simulink model "wlan_phy_tx_pmd"  (Simulink 7.8)
settings: Solver=ode45  StartTime=0.0  StopTime=17e3  RelTol=1e-3
PostLoadFcn:
  | wlan_phy_tx_init
InitFcn:
  | wlan_phy_tx_init
StartFcn:
  | wlan_phy_tx_init
undefined symbols (not defined in the file): gcbh, interleave_16QAM, interleave_64QAM_addr, interleave_bpsk, interleave_QPSK, MAX_NUM_BYTES, MAX_NUM_SC, Mod_Constellation_16QAM, Mod_Constellation_64QAM, Mod_Constellation_BPSK, Mod_Constellation_QPSK, Preamble_IQ, xlBlockLoadCallback, xlGetNormalizedPeriod
libraries: xbsIndex_r4 x1164, xbsEDKLib_r4 x1
(part 3 of 8)

== system wlan_phy_tx_pmd/FFT ==
  Q in : Inport
  I in : Inport  Port=2
  data_in_tvalid : Inport  Port=3
  data_in_tlast : Inport  Port=4
  "Last sym " : Inport  Port=5
  FFT Core : Subsystem
  FFT In : Scope  NumInputPorts=5
      settings: TimeRange=10000  YMin=0~0~-1~-1~0  YMax=1~1~1~1~1
  FFT Last Sym : Scope  NumInputPorts=6
      settings: TimeRange=10000  YMin=0~0~-1~-1~-1~0  YMax=1~80~1~1~1~1  SaveName=ScopeData19
  FFT Out : Scope  NumInputPorts=6
      settings: TimeRange=10000  YMin=0~0~-1~-1~-1~0  YMax=1~80~1~1~1~1
  Gateway Out{,1..13,15..16} (16 alike) : xbsIndex_r4/Gateway Out  inherit_from_input=off  hdl_port=off  timing_constraint=None  locs_specified=off  LOCs={}  UseAsDAC=off  DACChannel='1'  block_type=gatewayout
  Logical : xbsIndex_r4/Logical  logical_function=AND  inputs=2  en=off  latency=0  precision=Full  arith_type=Unsigned  n_bits=16  bin_pt=0  align_bp=on  dbl_ovrd=off  block_type=logical
  S-R Latch2 : Subsystem
  valid only : Subsystem
  valid only1 : Subsystem
  data_in_tready : Outport
  I out : Outport  Port=2
  Q out : Outport  Port=3
  data_out_tvalid : Outport  Port=4
  Last sym : Outport  Port=5
  wires:
  Gateway Out7/1 -> FFT In/5  "tlast"
  valid only/1(Q) -> Gateway Out3/1
  Gateway Out3/1 -> FFT In/4  "valid I data"
  Gateway Out2/1 -> FFT In/3  "I data"
  Gateway Out1/1 -> FFT In/1  "tready"
  Gateway Out/1 -> FFT In/2  "tvalid"
  Gateway Out13/1 -> FFT Out/4  "valid I data"
  Gateway Out12/1 -> FFT Out/3  "I data"
  Gateway Out10/1 -> FFT Out/1  "tvalid"
  valid only1/1(Q) -> Gateway Out13/1
  Gateway Out11/1 -> FFT Out/2  "xk_index"
  "Last sym "/1 -> S-R Latch2/1(S), Gateway Out4/1
  S-R Latch2/1(Q) -> Logical/2, Gateway Out6/1
  Logical/1 -> Last sym/1, Gateway Out15/1, Gateway Out9/1
  [TX_RESET] -> S-R Latch2/2(R), Gateway Out5/1
  Gateway Out15/1 -> FFT Out/6  "Last sym"
  Gateway Out16/1 -> FFT Out/5  "tlast"
  FFT Core/1(data_in_tready) -> data_in_tready/1, Gateway Out1/1, valid only/1(ready)
  FFT Core/2(I out) -> I out/1, Gateway Out12/1, valid only1/1(D)
  FFT Core/3(Q out) -> Q out/1
  Q in/1 -> FFT Core/1(Q in)
  I in/1 -> FFT Core/2(I in), valid only/3(D), Gateway Out2/1
  FFT Core/4(data_out_tvalid) -> data_out_tvalid/1, Gateway Out10/1, valid only1/2(valid)
  data_in_tvalid/1 -> FFT Core/3(data_in_tvalid), Gateway Out/1, valid only/2(valid)
  data_in_tlast/1 -> FFT Core/4(data_in_tlast), Gateway Out7/1
  FFT Core/6(data_out_tlast) -> Gateway Out16/1, Logical/1, Gateway Out8/1
  FFT Core/5(data_xk_index) -> Gateway Out11/1
  Gateway Out4/1 -> FFT Last Sym/1
  Gateway Out5/1 -> FFT Last Sym/2
  Gateway Out6/1 -> FFT Last Sym/3
  Gateway Out8/1 -> FFT Last Sym/4
  Gateway Out9/1 -> FFT Last Sym/5

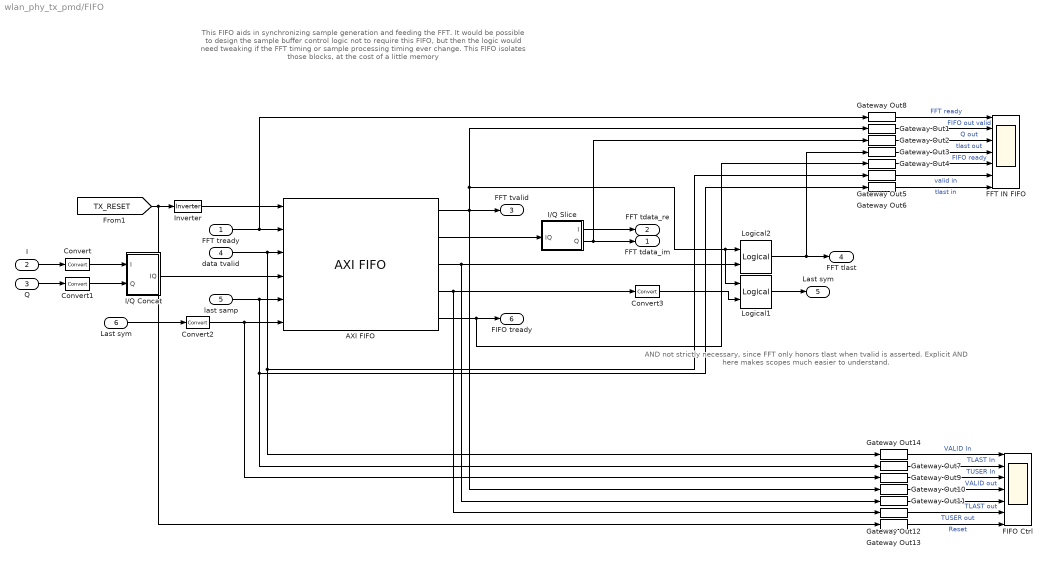
== system wlan_phy_tx_pmd/FIFO ==
  note: AND not strictly necessary, since FFT
      | only honors tlast when tvalid is asserted.
      | Explicit AND here makes scopes
      | much easier to understand.
  note: This FIFO aids in synchronizing sample generation
      | and feeding the FFT. It would be possible to design
      | the sample buffer control logic not to require
      | this FIFO, but then the logic would need tweaking
      | if the FFT timing or sample processing timing
      | ever change. This FIFO isolates those blocks,
      | at the cost of a little memory
  FFT tready : Inport
  I : Inport  Port=2
  Q : Inport  Port=3
  data tvalid : Inport  Port=4
  last samp : Inport  Port=5
  "Last sym " : Inport  Port=6
  AXI FIFO : xbsIndex_r4/AXI FIFO  input_depth_axis=64  actual_fifo_depth_label=66  enable_tdata=on  enable_tdest=off  enable_tstrb=off  enable_tready=on  enable_tid=off  enable_tuser=on  enable_tkeep=off  enable_tlast=on  has_aresetn=on  enable_data_counts_axis=off  fifo_implementation_type_axis=Common Clock Block RAM  trim_axipin_name=on  programmable_full_type_axis=Full  full_threshold_assert_value_axis=0  programmable_empty_type_axis=Empty  empty_threshold_assert_value_axis=1022  block_type=axi_fifo
  Convert : xbsIndex_r4/Convert  gui_display_data_type=Fixed-point  arith_type="Signed  (2's comp)"  n_bits=16  bin_pt=15  float_type=Single  exp_bits=8  fraction_bits=24  quantization=Truncate  overflow=Wrap  en=off  latency=0  dbl_ovrd=off  pipeline=off  block_type=convert
  Convert1 : xbsIndex_r4/Convert  gui_display_data_type=Fixed-point  arith_type="Signed  (2's comp)"  n_bits=16  bin_pt=15  float_type=Single  exp_bits=8  fraction_bits=24  quantization=Truncate  overflow=Wrap  en=off  latency=0  dbl_ovrd=off  pipeline=off  block_type=convert
  Convert2 : xbsIndex_r4/Convert  gui_display_data_type=Fixed-point  arith_type=Unsigned  n_bits=1  bin_pt=0  float_type=Single  exp_bits=8  fraction_bits=24  quantization=Truncate  overflow=Wrap  en=off  latency=0  dbl_ovrd=off  pipeline=off  block_type=convert
  Convert3 : xbsIndex_r4/Convert  gui_display_data_type=Boolean  arith_type=Boolean  n_bits=1  bin_pt=0  float_type=Single  exp_bits=8  fraction_bits=24  quantization=Truncate  overflow=Wrap  en=off  latency=0  dbl_ovrd=off  pipeline=off  block_type=convert
  FFT IN FIFO : Scope  NumInputPorts=7
      settings: TimeRange=30000  YMin=0~0~0~-0.1~0~-0.1~-0.1  YMax=300~300~1~1.1~4000~1.1~1.1  SaveName=ScopeData20
  FIFO Ctrl : Scope  NumInputPorts=7
      settings: TimeRange=30000  YMin=0~0~0~-0.1~-0.1~-0.1~-0.1  YMax=300~300~1~1.1~1.1~1.1~1.1  SaveName=ScopeData21
  Gateway Out{1..14} (14 alike) : xbsIndex_r4/Gateway Out  inherit_from_input=off  hdl_port=off  timing_constraint=None  locs_specified=off  LOCs={}  UseAsDAC=off  DACChannel='1'  block_type=gatewayout
  I/Q Concat : Subsystem
  I/Q Slice : Subsystem
  Inverter : xbsIndex_r4/Inverter  en=off  latency=0  dbl_ovrd=off  block_type=inv
  Logical1 : xbsIndex_r4/Logical  logical_function=AND  inputs=2  en=off  latency=0  precision=Full  arith_type=Unsigned  n_bits=16  bin_pt=0  align_bp=on  dbl_ovrd=off  block_type=logical
  Logical2 : xbsIndex_r4/Logical  logical_function=AND  inputs=2  en=off  latency=0  precision=Full  arith_type=Unsigned  n_bits=16  bin_pt=0  align_bp=on  dbl_ovrd=off  block_type=logical
  FFT tdata_im : Outport
  FFT tdata_re : Outport  Port=2
  FFT tvalid : Outport  Port=3
  FFT tlast : Outport  Port=4
  Last sym : Outport  Port=5
  FIFO tready : Outport  Port=6
  wires:
  FFT tready/1 -> Gateway Out8/1, AXI FIFO/2
  data tvalid/1 -> AXI FIFO/3, Gateway Out5/1, Gateway Out14/1
  last samp/1 -> AXI FIFO/5, Gateway Out6/1, Gateway Out7/1
  I/1 -> Convert/1
  Q/1 -> Convert1/1
  I/Q Concat/1(IQ) -> AXI FIFO/4
  [TX_RESET] -> Inverter/1, Gateway Out13/1
  Inverter/1 -> AXI FIFO/1
  Convert/1 -> I/Q Concat/1(I)
  Convert1/1 -> I/Q Concat/2(Q)
  "Last sym "/1 -> Convert2/1
  AXI FIFO/5 -> FIFO tready/1, Gateway Out4/1
  AXI FIFO/2 -> I/Q Slice/1(IQ)
  AXI FIFO/1 -> FFT tvalid/1, Gateway Out1/1, Logical2/1, Logical1/1, Gateway Out10/1
  AXI FIFO/3 -> Logical2/2, Gateway Out11/1
  Gateway Out8/1 -> FFT IN FIFO/1  "FFT ready"
  I/Q Slice/1(I) -> FFT tdata_re/1
  I/Q Slice/2(Q) -> FFT tdata_im/1, Gateway Out2/1
  Gateway Out1/1 -> FFT IN FIFO/2  "FIFO out valid"
  Gateway Out2/1 -> FFT IN FIFO/3  "Q out"
  Gateway Out3/1 -> FFT IN FIFO/4  "tlast out"
  Gateway Out4/1 -> FFT IN FIFO/5  "FIFO ready"
  Gateway Out5/1 -> FFT IN FIFO/6  "valid in"
  Gateway Out6/1 -> FFT IN FIFO/7  "tlast in"
  Logical2/1 -> FFT tlast/1, Gateway Out3/1
  AXI FIFO/4 -> Gateway Out12/1, Convert3/1
  Convert2/1 -> AXI FIFO/6, Gateway Out9/1
  Gateway Out14/1 -> FIFO Ctrl/1  "VALID In"
  Gateway Out7/1 -> FIFO Ctrl/2  "TLAST In"
  Gateway Out9/1 -> FIFO Ctrl/3  "TUSER In"
  Gateway Out10/1 -> FIFO Ctrl/4  "VALID out"
  Gateway Out11/1 -> FIFO Ctrl/5  "TLAST out"
  Gateway Out12/1 -> FIFO Ctrl/6  "TUSER out"
  Gateway Out13/1 -> FIFO Ctrl/7  "Reset"
  Logical1/1 -> Last sym/1
  Convert3/1 -> Logical1/2

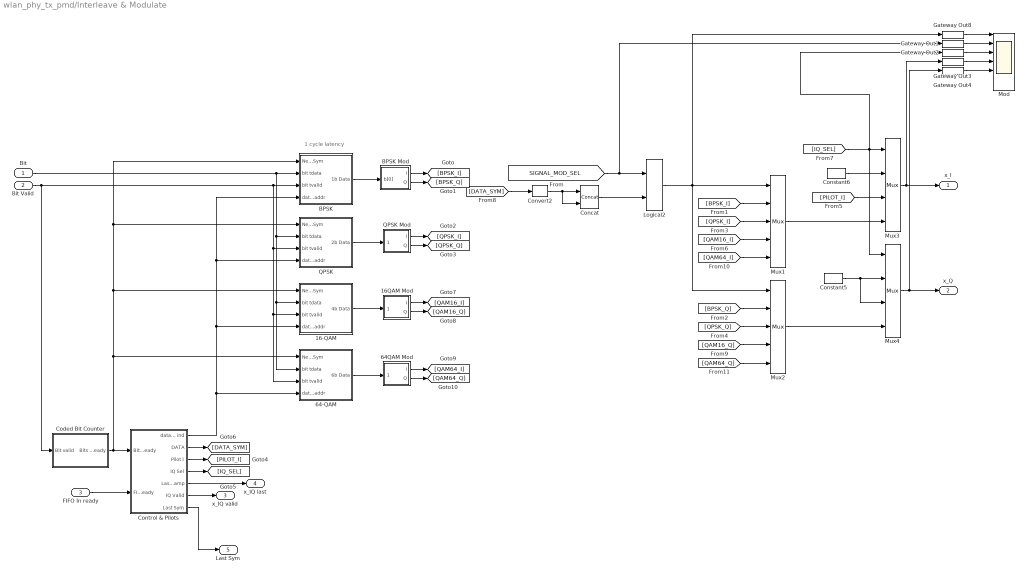
== system wlan_phy_tx_pmd/Interleave & Modulate ==
  note: 1 cycle latency
  Bit : Inport
  Bit Valid : Inport  Port=2
  FIFO In ready : Inport  Port=3
  16-QAM : Subsystem
  16QAM Mod : Subsystem
  64-QAM : Subsystem
  64QAM Mod : Subsystem
  BPSK : Subsystem
  BPSK Mod : Subsystem
  Coded Bit Counter : Subsystem
  Concat : xbsIndex_r4/Concat  num_inputs=2  dbl_ovrd=off  block_type=concat
  Constant5 : xbsIndex_r4/Constant  const=0  gui_display_data_type=Fixed-point  arith_type=Signed (2's comp)  n_bits=12  bin_pt=11  preci_type=Single  exp_width=8  frac_width=24  explicit_period=off  period=1  equ=P=C  opselect=C  inp2=PCIN>>17  opr=+  inp1=P  carry=CIN  dbl_ovrd=off  block_type=constant
  Constant6 : xbsIndex_r4/Constant  const=0  gui_display_data_type=Fixed-point  arith_type=Signed (2's comp)  n_bits=12  bin_pt=11  preci_type=Single  exp_width=8  frac_width=24  explicit_period=off  period=1  equ=P=C  opselect=C  inp2=PCIN>>17  opr=+  inp1=P  carry=CIN  dbl_ovrd=off  block_type=constant
  Control & Pilots : Subsystem
  Convert2 : xbsIndex_r4/Convert  gui_display_data_type=Fixed-point  arith_type=Unsigned  n_bits=1  bin_pt=0  float_type=Single  exp_bits=8  fraction_bits=24  quantization=Truncate  overflow=Wrap  en=off  latency=0  dbl_ovrd=off  pipeline=off  block_type=convert
  Gateway Out{1..4,8} (5 alike) : xbsIndex_r4/Gateway Out  inherit_from_input=off  hdl_port=off  timing_constraint=None  locs_specified=off  LOCs={}  UseAsDAC=off  DACChannel='1'  block_type=gatewayout
  Logical2 : xbsIndex_r4/Logical  logical_function=AND  inputs=2  en=off  latency=0  precision=Full  arith_type=Unsigned  n_bits=16  bin_pt=0  align_bp=on  dbl_ovrd=off  block_type=logical
  "Mod " : Scope  NumInputPorts=7
      settings: TimeRange=10000  YMin=0~0~0~-2~0~-0.1~-0.1  YMax=300~300~1~2~4000~1.1~1.1  SaveName=ScopeData7
  Mux1 : xbsIndex_r4/Mux  inputs=4  en=off  latency=0  precision=Full  arith_type=Unsigned  n_bits=16  bin_pt=14  quantization=Truncate  overflow=Wrap  dbl_ovrd=off  block_type=mux
  Mux2 : xbsIndex_r4/Mux  inputs=4  en=off  latency=0  precision=Full  arith_type=Unsigned  n_bits=16  bin_pt=14  quantization=Truncate  overflow=Wrap  dbl_ovrd=off  block_type=mux
  Mux3 : xbsIndex_r4/Mux  inputs=3  en=off  latency=0  precision=Full  arith_type=Unsigned  n_bits=16  bin_pt=14  quantization=Truncate  overflow=Wrap  dbl_ovrd=off  block_type=mux
  Mux4 : xbsIndex_r4/Mux  inputs=3  en=off  latency=0  precision=Full  arith_type=Unsigned  n_bits=16  bin_pt=14  quantization=Truncate  overflow=Wrap  dbl_ovrd=off  block_type=mux
  QPSK : Subsystem
  QPSK Mod : Subsystem
  x_I : Outport
  x_Q : Outport  Port=2
  x_IQ valid : Outport  Port=3
  x_IQ last : Outport  Port=4
  Last Sym : Outport  Port=5
  wires:
  Convert2/1 -> Concat/2, Concat/1
  [SIGNAL_MOD_SEL] -> Logical2/1, Gateway Out1/1
  Concat/1 -> Logical2/2
  Bit/1 -> BPSK/2("bit tdata "), QPSK/2("bit tdata "), 16-QAM/2("bit tdata "), 64-QAM/2("bit tdata ")
  Bit Valid/1 -> BPSK/3("bit tvalid "), QPSK/3("bit tvalid "), 16-QAM/3("bit tvalid "), 64-QAM/3("bit tvalid "), Coded Bit Counter/1(Bit valid)
  BPSK/1(1b Data) -> BPSK Mod/1(b[0])
  QPSK/1(2b Data) -> QPSK Mod/1(b[1:0])
  [QAM64_I] -> Mux1/5
  [QAM64_Q] -> Mux2/5
  BPSK Mod/1(I) -> [BPSK_I]
  BPSK Mod/2(Q) -> [BPSK_Q]
  QPSK Mod/1(I) -> [QPSK_I]
  QPSK Mod/2(Q) -> [QPSK_Q]
  [BPSK_Q] -> Mux2/2
  [BPSK_I] -> Mux1/2
  [QPSK_Q] -> Mux2/3
  Logical2/1 -> Mux1/1, Mux2/1, Gateway Out8/1
  [QPSK_I] -> Mux1/3
  Constant5/1 -> Mux4/2, Mux4/3
  Constant6/1 -> Mux3/2
  Control & Pilots/3(Pilot I) -> [PILOT_I]
  [PILOT_I] -> Mux3/3
  Mux1/1 -> Mux3/4
  Mux2/1 -> Mux4/4
  Mux3/1 -> x_I/1, Gateway Out3/1
  Mux4/1 -> x_Q/1, Gateway Out4/1
  Control & Pilots/4(IQ Sel) -> [IQ_SEL]
  [IQ_SEL] -> Mux3/1, Mux4/1, Gateway Out2/1
  Control & Pilots/5(Last Samp) -> x_IQ last/1
  Control & Pilots/6(IQ Valid) -> x_IQ valid/1
  [DATA_SYM] -> Convert2/1
  Control & Pilots/2(DATA) -> [DATA_SYM]
  Gateway Out8/1 -> "Mod "/1
  Gateway Out1/1 -> "Mod "/2
  Gateway Out2/1 -> "Mod "/3
  Gateway Out3/1 -> "Mod "/4
  Gateway Out4/1 -> "Mod "/5
  Coded Bit Counter/1(Bits Ready) -> Control & Pilots/1(Bits Ready), BPSK/1(New Sym), QPSK/1(New Sym), 16-QAM/1(New Sym), 64-QAM/1(New Sym)
  Control & Pilots/7(" Last Sym") -> Last Sym/1
  FIFO In ready/1 -> Control & Pilots/2(FIFO Ready)
  16-QAM/1(4b Data) -> 16QAM Mod/1(b[3:0])
  16QAM Mod/1(I) -> [QAM16_I]
  16QAM Mod/2(Q) -> [QAM16_Q]
  [QAM16_I] -> Mux1/4
  [QAM16_Q] -> Mux2/4
  Control & Pilots/1(data sym ind) -> 64-QAM/4(data sym addr), 16-QAM/4(data sym addr), QPSK/4(data sym addr), BPSK/4(data sym addr)
  64QAM Mod/1(I) -> [QAM64_I]
  64QAM Mod/2(Q) -> [QAM64_Q]
  64-QAM/1(6b Data) -> 64QAM Mod/1(b[5:0])

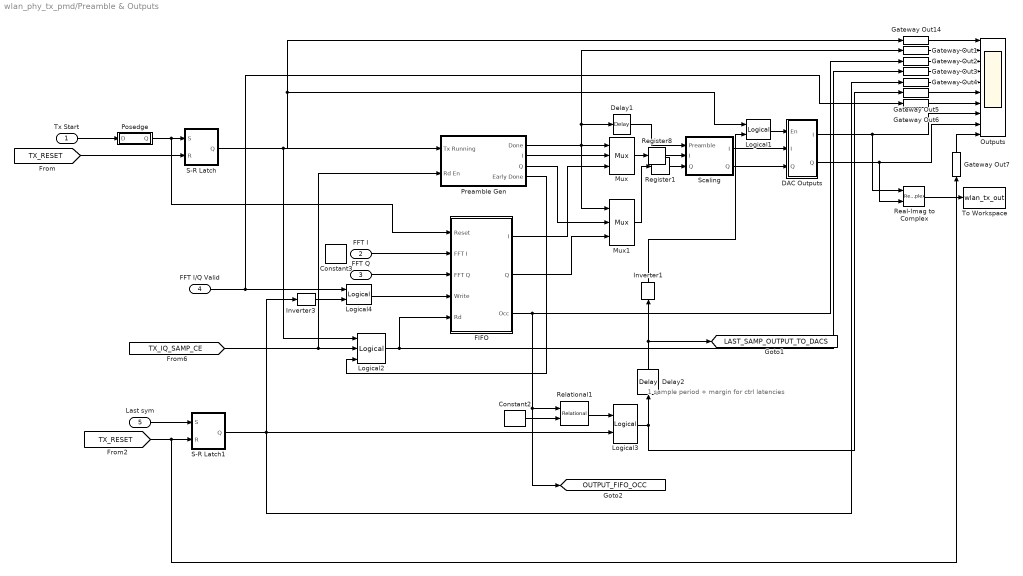
== system wlan_phy_tx_pmd/Preamble & Outputs ==
  note: 1 sample period + margin
      | for ctrl latencies
  Tx Start : Inport
  FFT I : Inport  Port=2
  FFT Q : Inport  Port=3
  FFT I/Q Valid : Inport  Port=4
  Last sym : Inport  Port=5
  Constant2 : xbsIndex_r4/Constant  const=0  gui_display_data_type=Fixed-point  arith_type=Unsigned  n_bits=1  bin_pt=0  preci_type=Single  exp_width=8  frac_width=24  explicit_period=off  period=1  equ=P=C  opselect=C  inp2=PCIN>>17  opr=+  inp1=P  carry=CIN  dbl_ovrd=off  block_type=constant
  Constant3 : xbsIndex_r4/Constant  const=-1  gui_display_data_type=Fixed-point  arith_type=Signed (2's comp)  n_bits=16  bin_pt=15  preci_type=Single  exp_width=8  frac_width=24  explicit_period=on  period=1  equ=P=C  opselect=C  inp2=PCIN>>17  opr=+  inp1=P  carry=CIN  dbl_ovrd=off  block_type=constant
  DAC Outputs : Subsystem
  Delay1 : xbsIndex_r4/Delay  rst=off  infoeditControl=Selection of Reset will increase slice count due to use of real FFs and instead of SRLs  en=off  latency=1  dbl_ovrd=off  reg_retiming=off  block_type=delay
  Delay2 : xbsIndex_r4/Delay  rst=off  infoeditControl=Selection of Reset will increase slice count due to use of real FFs and instead of SRLs  en=off  latency=12  dbl_ovrd=off  reg_retiming=off  block_type=delay
  FIFO : Subsystem
  Gateway Out{1..7,14} (8 alike) : xbsIndex_r4/Gateway Out  inherit_from_input=off  hdl_port=off  timing_constraint=None  locs_specified=off  LOCs={}  UseAsDAC=off  DACChannel='1'  block_type=gatewayout
  Inverter1 : xbsIndex_r4/Inverter  en=off  latency=0  dbl_ovrd=off  block_type=inv
      settings: xl_area=[0 0 0 0 0 0 0]  block_version=VER_STRING_GOES_HERE
  Inverter3 : xbsIndex_r4/Inverter  en=off  latency=0  dbl_ovrd=off  block_type=inv
      settings: xl_area=[0 0 0 0 0 0 0]  block_version=VER_STRING_GOES_HERE
  Logical1 : xbsIndex_r4/Logical  logical_function=AND  inputs=2  en=off  latency=0  precision=Full  arith_type=Unsigned  n_bits=16  bin_pt=0  align_bp=on  dbl_ovrd=off  block_type=logical
  Logical2 : xbsIndex_r4/Logical  logical_function=AND  inputs=3  en=off  latency=0  precision=Full  arith_type=Unsigned  n_bits=16  bin_pt=0  align_bp=on  dbl_ovrd=off  block_type=logical
  Logical3 : xbsIndex_r4/Logical  logical_function=AND  inputs=2  en=off  latency=0  precision=Full  arith_type=Unsigned  n_bits=16  bin_pt=0  align_bp=on  dbl_ovrd=off  block_type=logical
  Logical4 : xbsIndex_r4/Logical  logical_function=AND  inputs=2  en=off  latency=0  precision=Full  arith_type=Unsigned  n_bits=16  bin_pt=0  align_bp=on  dbl_ovrd=off  block_type=logical
  Mux : xbsIndex_r4/Mux  inputs=2  en=off  latency=0  precision=Full  arith_type=Unsigned  n_bits=16  bin_pt=14  quantization=Truncate  overflow=Wrap  dbl_ovrd=off  block_type=mux
  Mux1 : xbsIndex_r4/Mux  inputs=2  en=off  latency=0  precision=Full  arith_type=Unsigned  n_bits=16  bin_pt=14  quantization=Truncate  overflow=Wrap  dbl_ovrd=off  block_type=mux
  Outputs : Scope  NumInputPorts=10
      settings: TimeRange=12000  YMin=0~0~0~0~0~0~0~-1~-0.5~0  YMax=1~1~200~1~1~1~1~1~1~1  SaveName=ScopeData20
  Posedge : Subsystem
  Preamble Gen : Subsystem
  Real-Imag to Complex : RealImagToComplex
  Register1 : xbsIndex_r4/Register  init=0  rst=off  en=off  dbl_ovrd=off  block_type=register
  Register8 : xbsIndex_r4/Register  init=0  rst=off  en=off  dbl_ovrd=off  block_type=register
  Relational1 : xbsIndex_r4/Relational  mode=a=b  en=off  latency=0  dbl_ovrd=off  block_type=relational
  S-R Latch : Subsystem
  S-R Latch1 : Subsystem
  Scaling : Subsystem
  To Workspace : ToWorkspace  VariableName=wlan_tx_out  SampleTime=-1  SaveFormat=Array
      settings: Decimation=8
  tag scope: LAST_SAMP_OUTPUT_TO_DACS=global, OUTPUT_FIFO_OCC=global
  wires:
  Logical2/1 -> FIFO/5(Rd), Gateway Out3/1
  Posedge/1(Q) -> S-R Latch/1(S), FIFO/1(Reset)
  Tx Start/1 -> Posedge/1(D)
  [TX_RESET] -> S-R Latch/2(R)
  S-R Latch/1(Q) -> Logical2/1, Gateway Out14/1, Logical1/1, Preamble Gen/1(Tx Running)
  [TX_IQ_SAMP_CE] -> Logical2/2, Preamble Gen/2(Rd En)
  FFT Q/1 -> FIFO/3(FFT Q)
  Logical4/1 -> FIFO/4(Write)
  FIFO/3(" Occ") -> Relational1/1, [OUTPUT_FIFO_OCC], Gateway Out2/1
  Constant2/1 -> Relational1/2
  Relational1/1 -> Logical3/1
  Last sym/1 -> S-R Latch1/1(S)
  S-R Latch1/1(Q) -> Inverter3/1, Logical3/2, Gateway Out4/1
  Logical3/1 -> Gateway Out5/1, Delay2/1
  [TX_RESET] -> S-R Latch1/2(R), Gateway Out7/1
  Inverter3/1 -> Logical4/2
  FFT I/Q Valid/1 -> Logical4/1, Gateway Out6/1
  FIFO/1(" I") -> Mux/3
  DAC Outputs/1(" I") -> Real-Imag to Complex/1, Outputs/8
  Preamble Gen/2(I) -> Mux/2
  Gateway Out14/1 -> Outputs/1
  Gateway Out1/1 -> Outputs/2
  Gateway Out2/1 -> Outputs/3
  Gateway Out3/1 -> Outputs/4
  Gateway Out4/1 -> Outputs/5
  Gateway Out5/1 -> Outputs/6
  Preamble Gen/1(Done) -> Mux/1, Delay1/1, Gateway Out1/1, Mux1/1
  Real-Imag to Complex/1 -> To Workspace/1
  DAC Outputs/2(" Q") -> Real-Imag to Complex/2, Outputs/9
  Mux/1 -> Register8/1
  Mux1/1 -> Register1/1
  Preamble Gen/3(Q) -> Mux1/2
  FIFO/2(" Q") -> Mux1/3
  Scaling/1(" I") -> DAC Outputs/2(I)
  Scaling/2(" Q") -> DAC Outputs/3(Q)
  Delay1/1 -> Scaling/1(Preamble)
  Logical1/1 -> DAC Outputs/1(En)
  Inverter1/1 -> Logical1/2
  Delay2/1 -> Inverter1/1, [LAST_SAMP_OUTPUT_TO_DACS]
  Gateway Out6/1 -> Outputs/7
  Preamble Gen/4(Early Done) -> Logical2/3
  Gateway Out7/1 -> Outputs/10
  FFT I/1 -> FIFO/2(FFT I)
  Register8/1 -> Scaling/2(I)
  Register1/1 -> Scaling/3(Q)

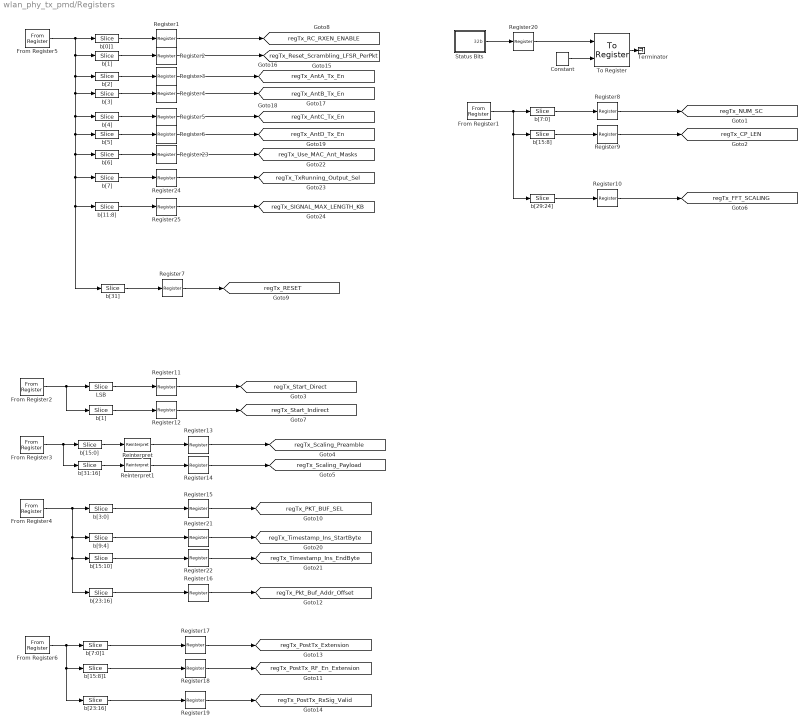
== system wlan_phy_tx_pmd/Registers ==
  Constant : xbsIndex_r4/Constant  const=1  gui_display_data_type=Boolean  arith_type=Boolean  n_bits=16  bin_pt=14  preci_type=Single  exp_width=8  frac_width=24  explicit_period=on  period=1  equ=P=C  opselect=C  inp2=PCIN>>17  opr=+  inp1=P  carry=CIN  dbl_ovrd=off  block_type=constant
  From Register1 : xbsIndex_r4/From Register  shared_memory_name='FFT_Config'  init=REG_TX_FFT_Config  period=1  ownership=Locally owned and initialized  gui_display_data_type=Fixed-point  arith_type=Unsigned  n_bits=32  bin_pt=0  preci_type=Single  dbl_ovrd=off  block_type=fromreg
      settings: AttributesFormatString=<< %<shared_memory_name> >>  infoedit="Register block that reads data to a shared memory register.  Delay of one sample period."
  From Register2 : xbsIndex_r4/From Register  shared_memory_name='TX_START'  init=0  period=1  ownership=Locally owned and initialized  gui_display_data_type=Fixed-point  arith_type=Unsigned  n_bits=32  bin_pt=0  preci_type=Single  dbl_ovrd=off  block_type=fromreg
      settings: AttributesFormatString=<< %<shared_memory_name> >>  infoedit="Register block that reads data to a shared memory register.  Delay of one sample period."
  From Register3 : xbsIndex_r4/From Register  shared_memory_name='Output_Scaling'  init=REG_TX_Output_Scaling  period=1  ownership=Locally owned and initialized  gui_display_data_type=Fixed-point  arith_type=Unsigned  n_bits=32  bin_pt=0  preci_type=Single  dbl_ovrd=off  block_type=fromreg
      settings: AttributesFormatString=<< %<shared_memory_name> >>  infoedit="Register block that reads data to a shared memory register.  Delay of one sample period."
  From Register4 : xbsIndex_r4/From Register  shared_memory_name='PKT_BUF_SEL'  init=REG_TX_PKT_BUF_SEL  period=1  ownership=Locally owned and initialized  gui_display_data_type=Fixed-point  arith_type=Unsigned  n_bits=32  bin_pt=0  preci_type=Single  dbl_ovrd=off  block_type=fromreg
      settings: AttributesFormatString=<< %<shared_memory_name> >>  infoedit="Register block that reads data to a shared memory register.  Delay of one sample period."
  From Register5 : xbsIndex_r4/From Register  shared_memory_name='Config'  init=REG_TX_Config  period=1  ownership=Locally owned and initialized  gui_display_data_type=Fixed-point  arith_type=Unsigned  n_bits=32  bin_pt=0  preci_type=Single  dbl_ovrd=off  block_type=fromreg
      settings: AttributesFormatString=<< %<shared_memory_name> >>  infoedit="Register block that reads data to a shared memory register.  Delay of one sample period."
  From Register6 : xbsIndex_r4/From Register  shared_memory_name='Timing'  init=REG_Tx_Timing  period=1  ownership=Locally owned and initialized  gui_display_data_type=Fixed-point  arith_type=Unsigned  n_bits=32  bin_pt=0  preci_type=Single  dbl_ovrd=off  block_type=fromreg
      settings: AttributesFormatString=<< %<shared_memory_name> >>  infoedit="Register block that reads data to a shared memory register.  Delay of one sample period."
  LSB : xbsIndex_r4/Slice  nbits=1  boolean_output=off  mode=Lower Bit Location + Width  bit1=0  base1=MSB of Input  bit0=0  base0=LSB of Input  dbl_ovrd=off  block_type=slice
      settings: block_version=VER_STRING_GOES_HERE
  Register{1..25} (25 alike) : xbsIndex_r4/Register  init=0  rst=off  en=off  dbl_ovrd=off  block_type=register
  Reinterpret : xbsIndex_r4/Reinterpret  force_arith_type=on  arith_type=Unsigned  force_bin_pt=on  bin_pt=12  block_type=reinterpret
  Reinterpret1 : xbsIndex_r4/Reinterpret  force_arith_type=on  arith_type=Unsigned  force_bin_pt=on  bin_pt=12  block_type=reinterpret
  Status Bits : Subsystem
  Terminator : Terminator
  To Register : xbsIndex_r4/To Register  shared_memory_name='STATUS'  init=0  ownership=Locally owned and initialized  explicit_data_type=on  gui_display_data_type=Fixed-point  arith_type=Unsigned  n_bits=32  bin_pt=0  preci_type=Single  dbl_ovrd=off  block_type=toreg
      settings: AttributesFormatString=<< %<shared_memory_name> >>  infoedit="Register block that writes data to a shared memory register.  Delay of one sample period."
  b[0]1 : xbsIndex_r4/Slice  nbits=1  boolean_output=off  mode=Lower Bit Location + Width  bit1=0  base1=MSB of Input  bit0=0  base0=LSB of Input  dbl_ovrd=off  block_type=slice
      settings: block_version=VER_STRING_GOES_HERE
  b[11:8] : xbsIndex_r4/Slice  nbits=4  boolean_output=off  mode=Lower Bit Location + Width  bit1=0  base1=MSB of Input  bit0=8  base0=LSB of Input  dbl_ovrd=off  block_type=slice
      settings: block_version=VER_STRING_GOES_HERE
  b[15:0] : xbsIndex_r4/Slice  nbits=16  boolean_output=off  mode=Lower Bit Location + Width  bit1=0  base1=MSB of Input  bit0=0  base0=LSB of Input  dbl_ovrd=off  block_type=slice
      settings: block_version=VER_STRING_GOES_HERE
  b[15:10] : xbsIndex_r4/Slice  nbits=6  boolean_output=off  mode=Lower Bit Location + Width  bit1=0  base1=MSB of Input  bit0=10  base0=LSB of Input  dbl_ovrd=off  block_type=slice
      settings: block_version=VER_STRING_GOES_HERE
  b[15:8] : xbsIndex_r4/Slice  nbits=8  boolean_output=off  mode=Lower Bit Location + Width  bit1=0  base1=MSB of Input  bit0=8  base0=LSB of Input  dbl_ovrd=off  block_type=slice
      settings: block_version=VER_STRING_GOES_HERE
  b[15:8]1 : xbsIndex_r4/Slice  nbits=8  boolean_output=off  mode=Lower Bit Location + Width  bit1=0  base1=MSB of Input  bit0=8  base0=LSB of Input  dbl_ovrd=off  block_type=slice
      settings: block_version=VER_STRING_GOES_HERE
  b[1] : xbsIndex_r4/Slice  nbits=1  boolean_output=on  mode=Lower Bit Location + Width  bit1=0  base1=MSB of Input  bit0=1  base0=LSB of Input  dbl_ovrd=off  block_type=slice
      settings: block_version=VER_STRING_GOES_HERE
  "b[1]  " : xbsIndex_r4/Slice  nbits=1  boolean_output=off  mode=Lower Bit Location + Width  bit1=0  base1=MSB of Input  bit0=1  base0=LSB of Input  dbl_ovrd=off  block_type=slice
      settings: block_version=VER_STRING_GOES_HERE
  b[23:16] : xbsIndex_r4/Slice  nbits=8  boolean_output=off  mode=Lower Bit Location + Width  bit1=0  base1=MSB of Input  bit0=16  base0=LSB of Input  dbl_ovrd=off  block_type=slice
      settings: block_version=VER_STRING_GOES_HERE
  "b[23:16] " : xbsIndex_r4/Slice  nbits=8  boolean_output=off  mode=Lower Bit Location + Width  bit1=0  base1=MSB of Input  bit0=16  base0=LSB of Input  dbl_ovrd=off  block_type=slice
      settings: block_version=VER_STRING_GOES_HERE
  b[29:24] : xbsIndex_r4/Slice  nbits=6  boolean_output=off  mode=Lower Bit Location + Width  bit1=0  base1=MSB of Input  bit0=24  base0=LSB of Input  dbl_ovrd=off  block_type=slice
      settings: block_version=VER_STRING_GOES_HERE
  b[2] : xbsIndex_r4/Slice  nbits=1  boolean_output=on  mode=Lower Bit Location + Width  bit1=0  base1=MSB of Input  bit0=2  base0=LSB of Input  dbl_ovrd=off  block_type=slice
      settings: block_version=VER_STRING_GOES_HERE
  b[31:16] : xbsIndex_r4/Slice  nbits=16  boolean_output=off  mode=Lower Bit Location + Width  bit1=0  base1=MSB of Input  bit0=16  base0=LSB of Input  dbl_ovrd=off  block_type=slice
      settings: block_version=VER_STRING_GOES_HERE
  b[31] : xbsIndex_r4/Slice  nbits=1  boolean_output=off  mode=Lower Bit Location + Width  bit1=0  base1=MSB of Input  bit0=31  base0=LSB of Input  dbl_ovrd=off  block_type=slice
      settings: block_version=VER_STRING_GOES_HERE
  b[3:0] : xbsIndex_r4/Slice  nbits=4  boolean_output=off  mode=Lower Bit Location + Width  bit1=0  base1=MSB of Input  bit0=0  base0=LSB of Input  dbl_ovrd=off  block_type=slice
      settings: block_version=VER_STRING_GOES_HERE
  b[3] : xbsIndex_r4/Slice  nbits=1  boolean_output=on  mode=Lower Bit Location + Width  bit1=0  base1=MSB of Input  bit0=3  base0=LSB of Input  dbl_ovrd=off  block_type=slice
      settings: block_version=VER_STRING_GOES_HERE
  b[4] : xbsIndex_r4/Slice  nbits=1  boolean_output=on  mode=Lower Bit Location + Width  bit1=0  base1=MSB of Input  bit0=4  base0=LSB of Input  dbl_ovrd=off  block_type=slice
      settings: block_version=VER_STRING_GOES_HERE
  b[5] : xbsIndex_r4/Slice  nbits=1  boolean_output=on  mode=Lower Bit Location + Width  bit1=0  base1=MSB of Input  bit0=5  base0=LSB of Input  dbl_ovrd=off  block_type=slice
      settings: block_version=VER_STRING_GOES_HERE
  b[6] : xbsIndex_r4/Slice  nbits=1  boolean_output=on  mode=Lower Bit Location + Width  bit1=0  base1=MSB of Input  bit0=6  base0=LSB of Input  dbl_ovrd=off  block_type=slice
      settings: block_version=VER_STRING_GOES_HERE
  b[7:0] : xbsIndex_r4/Slice  nbits=8  boolean_output=off  mode=Lower Bit Location + Width  bit1=0  base1=MSB of Input  bit0=0  base0=LSB of Input  dbl_ovrd=off  block_type=slice
      settings: block_version=VER_STRING_GOES_HERE
  b[7:0]1 : xbsIndex_r4/Slice  nbits=8  boolean_output=off  mode=Lower Bit Location + Width  bit1=0  base1=MSB of Input  bit0=0  base0=LSB of Input  dbl_ovrd=off  block_type=slice
      settings: block_version=VER_STRING_GOES_HERE
  b[7] : xbsIndex_r4/Slice  nbits=1  boolean_output=on  mode=Lower Bit Location + Width  bit1=0  base1=MSB of Input  bit0=7  base0=LSB of Input  dbl_ovrd=off  block_type=slice
      settings: block_version=VER_STRING_GOES_HERE
  b[9:4] : xbsIndex_r4/Slice  nbits=6  boolean_output=off  mode=Lower Bit Location + Width  bit1=0  base1=MSB of Input  bit0=4  base0=LSB of Input  dbl_ovrd=off  block_type=slice
      settings: block_version=VER_STRING_GOES_HERE
  tag scope: regTx_AntA_Tx_En=global, regTx_AntB_Tx_En=global, regTx_AntC_Tx_En=global, regTx_AntD_Tx_En=global, regTx_CP_LEN=global, regTx_FFT_SCALING=global, regTx_NUM_SC=global, regTx_PKT_BUF_SEL=global, regTx_Pkt_Buf_Addr_Offset=global, regTx_PostTx_Extension=global, regTx_PostTx_RF_En_Extension=global, regTx_PostTx_RxSig_Valid=global, regTx_RC_RXEN_ENABLE=global, regTx_RESET=global, regTx_Reset_Scrambling_LFSR_PerPkt=global, regTx_SIGNAL_MAX_LENGTH_KB=global, regTx_Scaling_Payload=global, regTx_Scaling_Preamble=global, regTx_Start_Direct=global, regTx_Start_Indirect=global, regTx_Timestamp_Ins_EndByte=global, regTx_Timestamp_Ins_StartByte=global, regTx_TxRunning_Output_Sel=global, regTx_Use_MAC_Ant_Masks=global
  wires:
  From Register5/1 -> b[0]1/1, b[1]/1, b[2]/1, b[3]/1, b[4]/1, b[5]/1, b[6]/1, b[7]/1, b[31]/1, b[11:8]/1
  From Register1/1 -> b[7:0]/1, b[15:8]/1, b[29:24]/1
  b[7:0]/1 -> Register8/1
  b[15:8]/1 -> Register9/1
  b[29:24]/1 -> Register10/1
  From Register2/1 -> LSB/1, "b[1]  "/1
  LSB/1 -> Register11/1
  From Register3/1 -> b[15:0]/1, b[31:16]/1
  b[15:0]/1 -> Reinterpret/1
  b[31:16]/1 -> Reinterpret1/1
  Reinterpret/1 -> Register13/1
  Reinterpret1/1 -> Register14/1
  "b[1]  "/1 -> Register12/1
  b[0]1/1 -> Register1/1
  b[31]/1 -> Register7/1
  Constant/1 -> To Register/2
  Status Bits/1(32b) -> Register20/1
  To Register/1 -> Terminator/1
  From Register4/1 -> b[3:0]/1, "b[23:16] "/1, b[15:10]/1, b[9:4]/1
  b[3:0]/1 -> Register15/1
  "b[23:16] "/1 -> Register16/1
  From Register6/1 -> b[7:0]1/1, b[15:8]1/1, b[23:16]/1
  b[7:0]1/1 -> Register17/1
  b[15:8]1/1 -> Register18/1
  b[23:16]/1 -> Register19/1
  b[1]/1 -> Register2/1
  b[2]/1 -> Register3/1
  b[3]/1 -> Register4/1
  b[4]/1 -> Register5/1
  b[5]/1 -> Register6/1
  Register1/1 -> [regTx_RC_RXEN_ENABLE]
  Register2/1 -> [regTx_Reset_Scrambling_LFSR_PerPkt]
  Register3/1 -> [regTx_AntA_Tx_En]
  Register4/1 -> [regTx_AntB_Tx_En]
  Register5/1 -> [regTx_AntC_Tx_En]
  Register6/1 -> [regTx_AntD_Tx_En]
  Register7/1 -> [regTx_RESET]
  Register8/1 -> [regTx_NUM_SC]
  Register9/1 -> [regTx_CP_LEN]
  Register10/1 -> [regTx_FFT_SCALING]
  Register11/1 -> [regTx_Start_Direct]
  Register12/1 -> [regTx_Start_Indirect]
  Register13/1 -> [regTx_Scaling_Preamble]
  Register14/1 -> [regTx_Scaling_Payload]
  Register15/1 -> [regTx_PKT_BUF_SEL]
  Register16/1 -> [regTx_Pkt_Buf_Addr_Offset]
  Register17/1 -> [regTx_PostTx_Extension]
  Register18/1 -> [regTx_PostTx_RF_En_Extension]
  Register19/1 -> [regTx_PostTx_RxSig_Valid]
  Register20/1 -> To Register/1
  b[9:4]/1 -> Register21/1
  Register21/1 -> [regTx_Timestamp_Ins_StartByte]
  b[15:10]/1 -> Register22/1
  Register22/1 -> [regTx_Timestamp_Ins_EndByte]
  b[6]/1 -> Register23/1
  Register23/1 -> [regTx_Use_MAC_Ant_Masks]
  b[11:8]/1 -> Register25/1
  Register25/1 -> [regTx_SIGNAL_MAX_LENGTH_KB]
  b[7]/1 -> Register24/1
  Register24/1 -> [regTx_TxRunning_Output_Sel]

== system wlan_phy_tx_pmd/Resets ==
  Constant : xbsIndex_r4/Constant  const=0  gui_display_data_type=Boolean  arith_type=Boolean  n_bits=16  bin_pt=14  preci_type=Single  exp_width=8  frac_width=24  explicit_period=on  period=1  equ=P=C  opselect=C  inp2=PCIN>>17  opr=+  inp1=P  carry=CIN  dbl_ovrd=off  block_type=constant
  Convert1 : xbsIndex_r4/Convert  gui_display_data_type=Boolean  arith_type=Boolean  n_bits=16  bin_pt=14  float_type=Single  exp_bits=8  fraction_bits=24  quantization=Truncate  overflow=Wrap  en=off  latency=0  dbl_ovrd=off  pipeline=off  block_type=convert
  Delay : xbsIndex_r4/Delay  rst=off  infoeditControl=Selection of Reset will increase slice count due to use of real FFs and instead of SRLs  en=off  latency=16  dbl_ovrd=off  reg_retiming=off  block_type=delay
  Gateway Out1 : xbsIndex_r4/Gateway Out  inherit_from_input=off  hdl_port=off  timing_constraint=None  locs_specified=off  LOCs={}  UseAsDAC=off  DACChannel='1'  block_type=gatewayout
  Gateway Out2 : xbsIndex_r4/Gateway Out  inherit_from_input=off  hdl_port=off  timing_constraint=None  locs_specified=off  LOCs={}  UseAsDAC=off  DACChannel='1'  block_type=gatewayout
  Gateway Out3 : xbsIndex_r4/Gateway Out  inherit_from_input=off  hdl_port=off  timing_constraint=None  locs_specified=off  LOCs={}  UseAsDAC=off  DACChannel='1'  block_type=gatewayout
  Logical : xbsIndex_r4/Logical  logical_function=OR  inputs=3  en=off  latency=0  precision=Full  arith_type=Unsigned  n_bits=16  bin_pt=0  align_bp=on  dbl_ovrd=off  block_type=logical
  Logical1 : xbsIndex_r4/Logical  logical_function=OR  inputs=2  en=off  latency=0  precision=Full  arith_type=Unsigned  n_bits=16  bin_pt=0  align_bp=on  dbl_ovrd=off  block_type=logical
  Posedge1 : Subsystem
  Resets : Scope  NumInputPorts=7
      settings: TimeRange=10000  YMin=0~0~0~-0.1~0~-0.1~-0.1  YMax=1~1~1~1.1~25~1.1~1.1  SaveName=ScopeData18
  S-R Latch : Subsystem
  Sim Reset : Subsystem
  Simulation Multiplexer : xbsIndex_r4/Simulation Multiplexer  sim_sel=1  hw_sel=2  block_type=simmux
      settings: infoedit="Distinguish input subsystems as \"simulation only\" and \"generation only\".  The input specified For Simulation will be used during Simulink simulation.  The input specified For Generation will be used during code generation.  This block will typically be used on the output of a HW Co-Simulation, Black Box, or ModelSim subsystem.<br><br>Hardware Notes: This block costs nothing."
  tag scope: TX_FORCE_RESET=global, TX_PHY_DONE=global, TX_RESET=global
  wires:
  S-R Latch/1(Q) -> Delay/1, Gateway Out2/1, Logical/3
  Logical/1 -> [TX_RESET], Gateway Out3/1
  Logical1/1 -> Posedge1/1(D)
  Delay/1 -> S-R Latch/2(R)
  Gateway Out1/1 -> Resets/2  "Last Samp Tx"
  Gateway Out2/1 -> Resets/3  "Last Samp SR"
  Gateway Out3/1 -> Resets/4  "TX_RESET"
  [regTx_RESET] -> Convert1/1
  Convert1/1 -> [TX_FORCE_RESET], Logical/2
  [LAST_SAMP_OUTPUT_TO_DACS] -> Logical1/1
  [SIGNAL_DECODE_ERROR] -> Logical1/2
  Posedge1/1(Q) -> S-R Latch/1(S), Gateway Out1/1, [TX_PHY_DONE]
  Simulation Multiplexer/1 -> Logical/1
  Constant/1 -> Simulation Multiplexer/2
  Sim Reset/1(Out1) -> Simulation Multiplexer/1

== system wlan_phy_tx_pmd/Scramble & Encode ==
  note: DATA and PAD are scrambled
      | SIGNAL and TAIL are not
  Bit : Inport
  Bit Valid : Inport  Port=2
  DATA/PAD/FCS : Inport  Port=3
  TAIL : Inport  Port=4
  Conv Enc : Subsystem
  Convert1 : xbsIndex_r4/Convert  gui_display_data_type=Fixed-point  arith_type=Unsigned  n_bits=1  bin_pt=0  float_type=Single  exp_bits=8  fraction_bits=24  quantization=Truncate  overflow=Wrap  en=off  latency=0  dbl_ovrd=off  pipeline=off  block_type=convert
  Convert2 : xbsIndex_r4/Convert  gui_display_data_type=Fixed-point  arith_type=Unsigned  n_bits=1  bin_pt=0  float_type=Single  exp_bits=8  fraction_bits=24  quantization=Truncate  overflow=Wrap  en=off  latency=0  dbl_ovrd=off  pipeline=off  block_type=convert
  Delay : xbsIndex_r4/Delay  rst=off  infoeditControl=Selection of Reset will increase slice count due to use of real FFs and instead of SRLs  en=off  latency=1  dbl_ovrd=off  reg_retiming=off  block_type=delay
  Delay1 : xbsIndex_r4/Delay  rst=off  infoeditControl=Selection of Reset will increase slice count due to use of real FFs and instead of SRLs  en=off  latency=2  dbl_ovrd=off  reg_retiming=off  block_type=delay
  Encoder : Scope  NumInputPorts=7
      settings: TimeRange=85.50254692050294  YMin=0~-0.1~-0.1~-0.1~-0.1~-0.1~-1  YMax=1~1.1~1.1~1.1~1.1~1.1~1  SaveName=ScopeData3
  Gateway Out{1..5,8} (6 alike) : xbsIndex_r4/Gateway Out  inherit_from_input=off  hdl_port=off  timing_constraint=None  locs_specified=off  LOCs={}  UseAsDAC=off  DACChannel='1'  block_type=gatewayout
  Inverter : xbsIndex_r4/Inverter  en=off  latency=0  dbl_ovrd=off  block_type=inv
  Logical : xbsIndex_r4/Logical  logical_function=XOR  inputs=2  en=off  latency=0  precision=Full  arith_type=Unsigned  n_bits=16  bin_pt=0  align_bp=on  dbl_ovrd=off  block_type=logical
  Logical1 : xbsIndex_r4/Logical  logical_function=AND  inputs=3  en=off  latency=0  precision=Full  arith_type=Unsigned  n_bits=16  bin_pt=0  align_bp=on  dbl_ovrd=off  block_type=logical
  Logical2 : xbsIndex_r4/Logical  logical_function=AND  inputs=2  en=off  latency=0  precision=Full  arith_type=Unsigned  n_bits=16  bin_pt=0  align_bp=on  dbl_ovrd=off  block_type=logical
  Mux : xbsIndex_r4/Mux  inputs=2  en=off  latency=0  precision=Full  arith_type=Unsigned  n_bits=16  bin_pt=14  quantization=Truncate  overflow=Wrap  dbl_ovrd=off  block_type=mux
  Puncture : Subsystem
  Scrambling LFSR : Subsystem
  Enc Bit : Outport
  Enc Bit Valid : Outport  Port=2
  wires:
  [TX_RESET] -> Conv Enc/1(Rst), Puncture/3(Reset)
  Mux/1 -> Enc Bit/1, Gateway Out3/1
  Logical/1 -> Conv Enc/3(Data), Gateway Out5/1
  Scrambling LFSR/1(Q) -> Logical1/2
  Logical1/1 -> Logical/2
  Convert1/1 -> Logical1/1
  DATA/PAD/FCS/1 -> Convert1/1, Puncture/1(DATA), Logical2/2, Gateway Out8/1
  Puncture/1(Coded Bit tvalid) -> Delay/1
  Logical2/1 -> Scrambling LFSR/1(en)
  Gateway Out8/1 -> Encoder/1  "DATA?"
  Gateway Out1/1 -> Encoder/3  "Bit In Valid"
  Gateway Out2/1 -> Encoder/4  "Enc Bit Sel"
  Gateway Out3/1 -> Encoder/5  "Enc Bit Out"
  Gateway Out4/1 -> Encoder/6  "Enc Bit Valid"
  TAIL/1 -> Inverter/1
  Inverter/1 -> Convert2/1
  Convert2/1 -> Logical1/3
  Gateway Out5/1 -> Encoder/2  "Data bit (scrambled)"
  Bit Valid/1 -> Logical2/1, Conv Enc/2(En), Puncture/2(Data Bit valid), Gateway Out1/1, Delay1/1
  Bit/1 -> Logical/1
  Conv Enc/1(A) -> Mux/2
  Conv Enc/2(B) -> Mux/3
  Delay/1 -> Enc Bit Valid/1, Gateway Out4/1
  Delay1/1 -> Mux/1, Gateway Out2/1

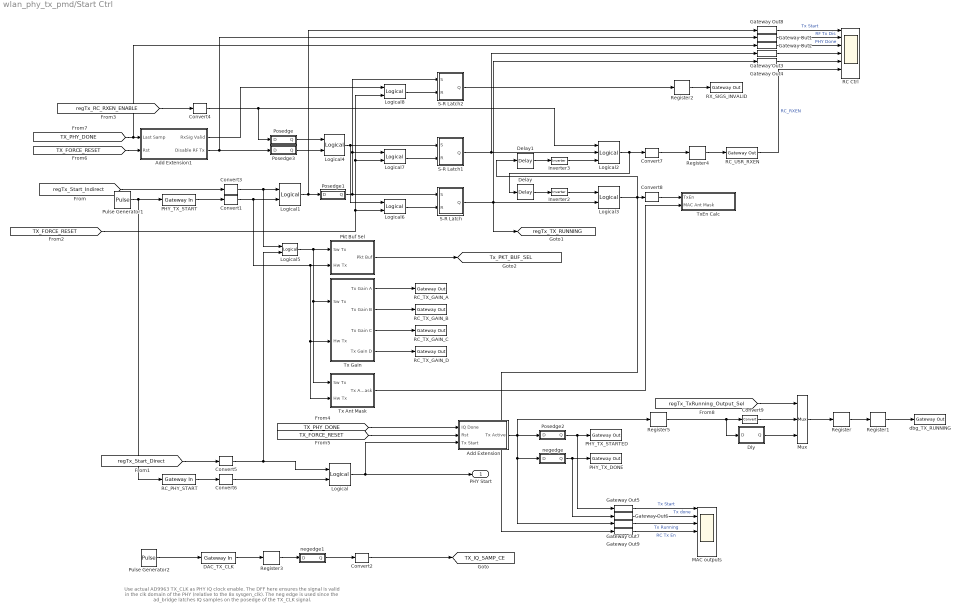
== system wlan_phy_tx_pmd/Start Ctrl ==
  note: Use actual AD9963 TX_CLK as PHY IQ clock enable.
      | The DFF here ensures the signal is valid in the clk
      | domain of the PHY (relative to the 8x sysgen_clk). The
      | neg edge is used since the ad_bridge latches IQ samples
      | on the posedge of the TX_CLK signal.
  Add Extension : Subsystem
  Add Extension1 : Subsystem
  Convert{1..6} (6 alike) : xbsIndex_r4/Convert  gui_display_data_type=Boolean  arith_type=Boolean  n_bits=1  bin_pt=0  float_type=Single  exp_bits=8  fraction_bits=24  quantization=Truncate  overflow=Wrap  en=off  latency=0  dbl_ovrd=off  pipeline=off  block_type=convert
  Convert7 : xbsIndex_r4/Convert  gui_display_data_type=Fixed-point  arith_type=Unsigned  n_bits=1  bin_pt=0  float_type=Single  exp_bits=8  fraction_bits=24  quantization=Truncate  overflow=Wrap  en=off  latency=0  dbl_ovrd=off  pipeline=off  block_type=convert
  Convert8 : xbsIndex_r4/Convert  gui_display_data_type=Fixed-point  arith_type=Unsigned  n_bits=1  bin_pt=0  float_type=Single  exp_bits=8  fraction_bits=24  quantization=Truncate  overflow=Wrap  en=off  latency=0  dbl_ovrd=off  pipeline=off  block_type=convert
  Convert9 : xbsIndex_r4/Convert  gui_display_data_type=Fixed-point  arith_type=Unsigned  n_bits=1  bin_pt=0  float_type=Single  exp_bits=8  fraction_bits=24  quantization=Truncate  overflow=Wrap  en=off  latency=0  dbl_ovrd=off  pipeline=off  block_type=convert
  DAC_TX_CLK : xbsIndex_r4/Gateway In  gui_display_data_type=Fixed-point  arith_type=Unsigned  n_bits=1  bin_pt=0  preci_type=Single  exp_width=8  frac_width=24  quantization="Round  (unbiased: +/- Inf)"  overflow=Saturate  period=1  dbl_ovrd=off  timing_constraint=None  locs_specified=off  LOCs={}  UseAsADC=off  ADCChannel='1'  inherit_from_input=off  hdl_port=on  block_type=gatewayin
  Delay : xbsIndex_r4/Delay  rst=off  infoeditControl=Selection of Reset will increase slice count due to use of real FFs and instead of SRLs  en=off  latency=32  dbl_ovrd=off  reg_retiming=off  block_type=delay
  Delay1 : xbsIndex_r4/Delay  rst=off  infoeditControl=Selection of Reset will increase slice count due to use of real FFs and instead of SRLs  en=off  latency=32  dbl_ovrd=off  reg_retiming=off  block_type=delay
  Dly : Subsystem
  Gateway Out{1..9} (9 alike) : xbsIndex_r4/Gateway Out  inherit_from_input=off  hdl_port=off  timing_constraint=None  locs_specified=off  LOCs={}  UseAsDAC=off  DACChannel='1'  block_type=gatewayout
  Inverter2 : xbsIndex_r4/Inverter  en=off  latency=0  dbl_ovrd=off  block_type=inv
  Inverter3 : xbsIndex_r4/Inverter  en=off  latency=0  dbl_ovrd=off  block_type=inv
  Logical{,1,4..8} (7 alike) : xbsIndex_r4/Logical  logical_function=OR  inputs=2  en=off  latency=0  precision=Full  arith_type=Unsigned  n_bits=16  bin_pt=0  align_bp=on  dbl_ovrd=off  block_type=logical
  Logical2 : xbsIndex_r4/Logical  logical_function=AND  inputs=3  en=off  latency=0  precision=Full  arith_type=Unsigned  n_bits=16  bin_pt=0  align_bp=on  dbl_ovrd=off  block_type=logical
  Logical3 : xbsIndex_r4/Logical  logical_function=AND  inputs=2  en=off  latency=0  precision=Full  arith_type=Unsigned  n_bits=16  bin_pt=0  align_bp=on  dbl_ovrd=off  block_type=logical
  MAC outputs : Scope  NumInputPorts=7
      settings: TimeRange=15000  YMin=0~0~0~0~0~0~0  YMax=1~1~1~1~1~1~1  SaveName=ScopeData25
  Mux : xbsIndex_r4/Mux  inputs=2  en=off  latency=0  precision=Full  arith_type=Unsigned  n_bits=16  bin_pt=14  quantization=Truncate  overflow=Wrap  dbl_ovrd=off  block_type=mux
  PHY_TX_DONE : xbsIndex_r4/Gateway Out  inherit_from_input=off  hdl_port=on  timing_constraint=None  locs_specified=off  LOCs={}  UseAsDAC=off  DACChannel='1'  block_type=gatewayout
  PHY_TX_START : xbsIndex_r4/Gateway In  gui_display_data_type=Fixed-point  arith_type=Unsigned  n_bits=1  bin_pt=0  preci_type=Single  exp_width=8  frac_width=24  quantization="Round  (unbiased: +/- Inf)"  overflow=Saturate  period=1  dbl_ovrd=off  timing_constraint=None  locs_specified=off  LOCs={}  UseAsADC=off  ADCChannel='1'  inherit_from_input=off  hdl_port=on  block_type=gatewayin
  PHY_TX_STARTED : xbsIndex_r4/Gateway Out  inherit_from_input=off  hdl_port=on  timing_constraint=None  locs_specified=off  LOCs={}  UseAsDAC=off  DACChannel='1'  block_type=gatewayout
  Pkt Buf Sel : Subsystem
  Posedge : Subsystem
  Posedge1 : Subsystem
  Posedge2 : Subsystem
  Posedge3 : Subsystem
  Pulse Generator1 : DiscretePulseGenerator  Period=8001  PhaseDelay=151
  Pulse Generator2 : DiscretePulseGenerator  Period=8  PulseWidth=4
  RC Ctrl : Scope  NumInputPorts=7
      settings: TimeRange=15000  YMin=0~0~0~0~0~0~0  YMax=1~1~1~1~1~1~1  SaveName=ScopeData22
  RC_PHY_START : xbsIndex_r4/Gateway In  gui_display_data_type=Fixed-point  arith_type=Unsigned  n_bits=1  bin_pt=0  preci_type=Single  exp_width=8  frac_width=24  quantization="Round  (unbiased: +/- Inf)"  overflow=Saturate  period=1  dbl_ovrd=off  timing_constraint=None  locs_specified=off  LOCs={}  UseAsADC=off  ADCChannel='1'  inherit_from_input=off  hdl_port=on  block_type=gatewayin
  RC_TX_GAIN_A : xbsIndex_r4/Gateway Out  inherit_from_input=off  hdl_port=on  timing_constraint=None  locs_specified=off  LOCs={}  UseAsDAC=off  DACChannel='1'  block_type=gatewayout
  RC_TX_GAIN_B : xbsIndex_r4/Gateway Out  inherit_from_input=off  hdl_port=on  timing_constraint=None  locs_specified=off  LOCs={}  UseAsDAC=off  DACChannel='1'  block_type=gatewayout
  RC_TX_GAIN_C : xbsIndex_r4/Gateway Out  inherit_from_input=off  hdl_port=on  timing_constraint=None  locs_specified=off  LOCs={}  UseAsDAC=off  DACChannel='1'  block_type=gatewayout
  RC_TX_GAIN_D : xbsIndex_r4/Gateway Out  inherit_from_input=off  hdl_port=on  timing_constraint=None  locs_specified=off  LOCs={}  UseAsDAC=off  DACChannel='1'  block_type=gatewayout
  RC_USR_RXEN : xbsIndex_r4/Gateway Out  inherit_from_input=off  hdl_port=on  timing_constraint=None  locs_specified=off  LOCs={}  UseAsDAC=off  DACChannel='1'  block_type=gatewayout
  RX_SIGS_INVALID : xbsIndex_r4/Gateway Out  inherit_from_input=off  hdl_port=on  timing_constraint=None  locs_specified=off  LOCs={}  UseAsDAC=off  DACChannel='1'  block_type=gatewayout
  Register{,1..5} (6 alike) : xbsIndex_r4/Register  init=0  rst=off  en=off  dbl_ovrd=off  block_type=register
  S-R Latch : Subsystem
  S-R Latch1 : Subsystem
  S-R Latch2 : Subsystem
  Tx Ant Mask : Subsystem
  Tx Gain : Subsystem
  TxEn Calc : Subsystem
  dbg_TX_RUNNING : xbsIndex_r4/Gateway Out  inherit_from_input=off  hdl_port=on  timing_constraint=None  locs_specified=off  LOCs={}  UseAsDAC=off  DACChannel='1'  block_type=gatewayout
  negedge : Subsystem
  negedge1 : Subsystem
  PHY Start : Outport
  tag scope: TX_IQ_SAMP_CE=global, Tx_PKT_BUF_SEL=global, regTx_TX_RUNNING=global
  wires:
  RC_PHY_START/1 -> Convert6/1
  Logical/1 -> PHY Start/1, Add Extension/3(Tx Start)
  [regTx_Start_Direct] -> Convert5/1
  S-R Latch/1(Q) -> Logical3/2, [regTx_TX_RUNNING], Gateway Out4/1
  Logical1/1 -> Posedge1/1(D), Gateway Out8/1
  PHY_TX_START/1 -> Convert1/1
  [regTx_Start_Indirect] -> Convert3/1
  S-R Latch1/1(Q) -> Logical2/2, Gateway Out3/1
  Logical2/1 -> Delay/1, Convert7/1
  [regTx_RC_RXEN_ENABLE] -> Convert4/1
  Inverter2/1 -> Logical3/1
  Delay/1 -> Inverter2/1
  Delay1/1 -> Inverter3/1
  Inverter3/1 -> Logical2/3
  Logical3/1 -> Delay1/1, Gateway Out9/1, Convert8/1
  Logical4/1 -> S-R Latch1/1(S), Logical6/1
  Posedge/1(Q) -> Logical4/1
  Posedge1/1(Q) -> S-R Latch/1(S), S-R Latch2/1(S), Logical7/1
  Gateway Out8/1 -> RC Ctrl/1  "Tx Start"
  Gateway Out1/1 -> RC Ctrl/2  "RF Tx Dis"
  Gateway Out2/1 -> RC Ctrl/3  "PHY Done"
  Gateway Out3/1 -> RC Ctrl/4
  Gateway Out4/1 -> RC Ctrl/5
  [TX_PHY_DONE] -> Add Extension/1(IQ Done)
  Add Extension/1(Tx Active) -> Posedge2/1(D), negedge/1(D), Gateway Out7/1, Register5/1
  [TX_FORCE_RESET] -> Add Extension/2(Rst)
  negedge/1(Q) -> PHY_TX_DONE/1, Gateway Out6/1
  Posedge2/1(Q) -> PHY_TX_STARTED/1, Gateway Out5/1
  Logical5/1 -> Pkt Buf Sel/1(Sw Tx), Tx Ant Mask/1(Sw Tx), Tx Gain/1(Sw Tx)
  Pkt Buf Sel/1(Pkt Buf) -> [Tx_PKT_BUF_SEL]
  Register/1 -> Register1/1
  Register1/1 -> dbg_TX_RUNNING/1
  Add Extension1/2(Disable RF Tx) -> Posedge3/1(D), Gateway Out1/1
  [TX_PHY_DONE] -> Add Extension1/1(Last Samp), Gateway Out2/1
  [TX_FORCE_RESET] -> Add Extension1/2(Rst)
  Posedge3/1(Q) -> Logical4/2
  Pulse Generator1/1 -> PHY_TX_START/1, RC_PHY_START/1
  S-R Latch2/1(Q) -> Register2/1
  Add Extension1/1(RxSig Valid) -> Logical8/1
  Register2/1 -> RX_SIGS_INVALID/1
  Gateway Out5/1 -> MAC outputs/1  "Tx Start"
  Gateway Out6/1 -> MAC outputs/2  "Tx done"
  Gateway Out7/1 -> MAC outputs/3  "Tx Running"
  Gateway Out9/1 -> MAC outputs/4  "RC Tx En"
  Pulse Generator2/1 -> DAC_TX_CLK/1
  DAC_TX_CLK/1 -> Register3/1
  negedge1/1(Q) -> Convert2/1
  Convert2/1 -> [TX_IQ_SAMP_CE]
  Register3/1 -> negedge1/1(D)
  Logical6/1 -> S-R Latch/2(R)
  Logical7/1 -> S-R Latch1/2(R)
  Logical8/1 -> S-R Latch2/2(R)
  [TX_FORCE_RESET] -> Logical6/2, Logical8/2, Logical7/2
  Convert1/1 -> Logical1/2, Pkt Buf Sel/2(Hw Tx), Tx Gain/2(Hw Tx), Tx Ant Mask/2(Hw Tx)
  Convert3/1 -> Logical1/1, Logical5/1
  Convert4/1 -> Logical2/1, Posedge/1(D)
  Convert5/1 -> Logical/1, Logical5/2
  Convert6/1 -> Logical/2
  Convert7/1 -> Register4/1
  Register4/1 -> RC_USR_RXEN/1
  Tx Gain/1(Tx Gain A) -> RC_TX_GAIN_A/1
  RC_USR_RXEN/1 -> RC Ctrl/6  "RC_RXEN"
  Convert8/1 -> TxEn Calc/1(TxEn)
  Tx Ant Mask/1(Tx Ant Mask) -> TxEn Calc/2(MAC Ant Mask)
  Tx Gain/2(Tx Gain B) -> RC_TX_GAIN_B/1
  Tx Gain/3(Tx Gain C) -> RC_TX_GAIN_C/1
  Tx Gain/4(Tx Gain D) -> RC_TX_GAIN_D/1
  Dly/1(Q) -> Mux/3
  [regTx_TxRunning_Output_Sel] -> Mux/1
  Mux/1 -> Register/1
  Register5/1 -> Dly/1(D), Convert9/1
  Convert9/1 -> Mux/2
